simulink model "Experiment_4_2_Controller"  (R2018a)
settings: Solver=VariableStepAuto  StartTime=0.0  StopTime=50  RelTol=1e-3  EnableMultiTasking=on
undefined symbols (not defined in the file or in its folder): Ts
libraries: EEE481Arduino x2
settings Model: ExtModeTrigDuration=2  Creator=abhig  LastModifiedBy=abhig
settings RTWCC: BuildConfiguration=Faster Runs

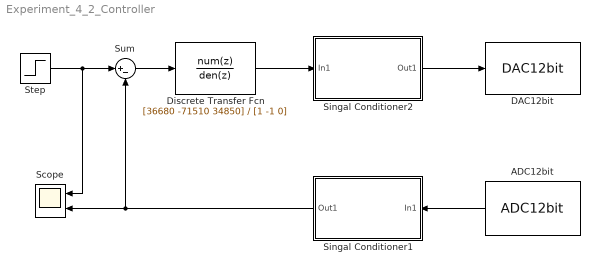
== system Experiment_4_2_Controller ==
  ADC12bit : EEE481Arduino/ADC12bit  pinNum=0  Tsa=Ts
      settings: SourceProductName=EEE 481 Arduino
  DAC12bit : EEE481Arduino/DAC12bit  Tsa=Ts  DACNum=0
      settings: SourceProductName=EEE 481 Arduino
  Discrete Transfer Fcn : DiscreteTransferFcn  Numerator=[36680 -71510 34850]  Denominator=[1 -1 0]
  Scope : Scope  NumInputPorts=2
  Singal Conditioner1 : Subsystem  mask{out_min=-pi/2, out_max=pi/2, in_min=0.56, in_max=2.76}
      mask prompts: out_min "Minimum Value of Output Signal"; out_max "Maximum Value of Output Signal"; in_min "Minimum Value of Input Signal"; in_max "Maximum Value of Input Signal"
  Singal Conditioner2 : Subsystem  mask{out_min=0.56, out_max=2.76, in_min=-255, in_max=255}
      mask prompts: out_min "Minimum Value of Output Signal"; out_max "Maximum Value of Output Signal"; in_min "Minimum Value of Input Signal"; in_max "Maximum Value of Input Signal"
  Step : Step  Time=25  After=pi/6  SampleTime=Ts
  Sum : Sum  Inputs=|+-
  wires:
  Singal Conditioner2/1(Out1) -> DAC12bit/1
  ADC12bit/1 -> Singal Conditioner1/1(In1)
  Discrete Transfer Fcn/1 -> Singal Conditioner2/1(In1)
  Sum/1 -> Discrete Transfer Fcn/1
  Singal Conditioner1/1(Out1) -> Scope/2, Sum/2
  Step/1 -> Scope/1, Sum/1

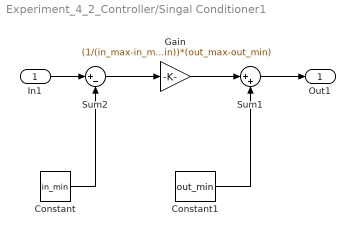
== system Experiment_4_2_Controller/Singal Conditioner1 ==
  In1 : Inport
  Constant : Constant  Value=in_min
  Constant1 : Constant  Value=out_min
  Gain : Gain  Gain=(1/(in_max-in_min))*(out_max-out_min)
  Sum1 : Sum  Inputs=|++
  Sum2 : Sum  Inputs=|+-
  Out1 : Outport
  wires:
  Constant/1 -> Sum2/2
  Gain/1 -> Sum1/1
  Sum1/1 -> Out1/1
  Constant1/1 -> Sum1/2
  In1/1 -> Sum2/1
  Sum2/1 -> Gain/1

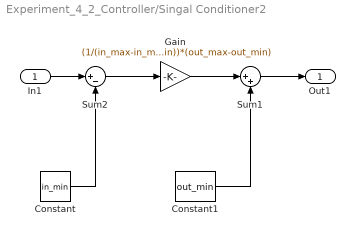
== system Experiment_4_2_Controller/Singal Conditioner2 ==
  In1 : Inport
  Constant : Constant  Value=in_min
  Constant1 : Constant  Value=out_min
  Gain : Gain  Gain=(1/(in_max-in_min))*(out_max-out_min)
  Sum1 : Sum  Inputs=|++
  Sum2 : Sum  Inputs=|+-
  Out1 : Outport
  wires:
  Sum2/1 -> Gain/1
  In1/1 -> Sum2/1
  Constant1/1 -> Sum1/2
  Sum1/1 -> Out1/1
  Gain/1 -> Sum1/1
  Constant/1 -> Sum2/2
